simulink model "ddc_bpm_476_066"  (Simulink 7.8)
settings: Solver=ode45  StartTime=0.0  StopTime=4e-4  RelTol=1e-3
undefined symbols (not defined in the file): dt_sim, frev_476, Fs_adc, xlipgetpartsetting
libraries: xbsIndex_r4 x515, simulink x3
(part 4 of 6)

== system ddc_bpm_476_066/Channel0_fofb/Analysis ==
  CIC_FOFB : Scope  NumInputPorts=2
      settings: TimeRange=0.00011214  YMin=-0.232331~-0.265937  YMax=-0.232331~-0.265937  SaveName=ScopeData4  MaxDataPoints=1000000  SampleInput=on
  CORDIC_FOFB : Scope  NumInputPorts=2
      settings: TimeRange=0.00011214  YMin=0.475054~-10  YMax=0.52506~45  SaveName=ScopeData5  MaxDataPoints=1000000  SampleInput=on
  bpf_ch0_o{5..8} (4 alike) : xbsIndex_r4/Gateway Out  inherit_from_input=on  hdl_port=off  timing_constraint=Data Rate  locs_specified=off  LOCs={}  UseAsDAC=off  DACChannel='1'  block_type=gatewayout
      settings: infoedit="Gateway out block.  Converts Xilinx fixed-point or floating-point type inputs into ouputs of type Simulink integer, single, double, or fixed point.<br><br>Hardware notes:  In hardware these blocks become top level output ports or are discarded, depending on how they are configured."
  wires:
  bpf_ch0_o5/1 -> CIC_FOFB/1
  [CIC_FOFB_I_FPGA_OUT] -> bpf_ch0_o5/1
  bpf_ch0_o6/1 -> CIC_FOFB/2
  [CIC_FOFB_Q_FPGA_OUT] -> bpf_ch0_o6/1
  bpf_ch0_o7/1 -> CORDIC_FOFB/1
  [CORDIC_FOFB_R_FPGA_OUT] -> bpf_ch0_o7/1
  bpf_ch0_o8/1 -> CORDIC_FOFB/2
  [CORDIC_FOFB_T_FPGA_OUT] -> bpf_ch0_o8/1

== system ddc_bpm_476_066/Channel0_fofb/cic_fofb ==
  Q_in : Inport
  I_in : Inport  Port=2
  Reinterpret : xbsIndex_r4/Reinterpret  force_arith_type=on  arith_type="Signed  (2's comp)"  force_bin_pt=on  bin_pt=23  block_type=reinterpret
  Reinterpret1 : xbsIndex_r4/Reinterpret  force_arith_type=on  arith_type="Signed  (2's comp)"  force_bin_pt=on  bin_pt=23  block_type=reinterpret
  Terminator : Terminator
  Terminator1 : Terminator
  cic_fofb_i : xbsIndex_r4/CIC Compiler 3.0   filter_type=Decimation  number_of_stages=5  differential_delay=2  number_of_channels=1  sample_rate_changes=Fixed  fixed_or_initial_rate=R_fofb  minimum_rate=1113  maximum_rate=1113  ratespecification=Maximum_Possible  sampleperiod=1  hardwareoversamplingrate=1  quantization=Truncation  output_data_width=25  use_xtreme_dsp_slice=on  use_streaming_interface=on  has_aclken=off  has_aresetn=off  has_dout_tready=off  trim_axipin_name=on  gui_behaviour=Sysgen_GUI  input_data_width=18  ip_name=CIC Compiler  ip_version=3.0  dsptool_ready=true  wrapper_available=true  port_translation_map={ 'aclken' => 'en', 'aresetn' => 'rst' }  ipcore_xco_need_fpga_part=true  ipcore_fpga_part=xlipgetpartsetting(gcb, {'virtex7', 'xc7v1500t', '-2', 'fhg1157'})  ipcore_verbose=false  block_type=cic_compiler_v3_0
  cic_fofb_q : xbsIndex_r4/CIC Compiler 3.0   filter_type=Decimation  number_of_stages=5  differential_delay=2  number_of_channels=1  sample_rate_changes=Fixed  fixed_or_initial_rate=R_fofb  minimum_rate=1113  maximum_rate=1113  ratespecification=Maximum_Possible  sampleperiod=1  hardwareoversamplingrate=1  quantization=Truncation  output_data_width=25  use_xtreme_dsp_slice=on  use_streaming_interface=on  has_aclken=off  has_aresetn=off  has_dout_tready=off  trim_axipin_name=on  gui_behaviour=Sysgen_GUI  input_data_width=18  ip_name=CIC Compiler  ip_version=3.0  dsptool_ready=true  wrapper_available=true  port_translation_map={ 'aclken' => 'en', 'aresetn' => 'rst' }  ipcore_xco_need_fpga_part=true  ipcore_fpga_part=xlipgetpartsetting(gcb, {'virtex7', 'xc7v1500t', '-2', 'fhg1157'})  ipcore_verbose=false  block_type=cic_compiler_v3_0
  Q_out : Outport
  Q_valid : Outport  Port=2
  I_out : Outport  Port=3
  I_valid : Outport  Port=4
  wires:
  I_in/1 -> cic_fofb_i/1
  cic_fofb_i/2 -> I_valid/1
  Q_in/1 -> cic_fofb_q/1
  cic_fofb_q/2 -> Q_valid/1
  cic_fofb_i/1 -> Terminator/1
  cic_fofb_q/1 -> Terminator1/1
  Reinterpret/1 -> Q_out/1
  cic_fofb_q/3 -> Reinterpret/1
  Reinterpret1/1 -> I_out/1
  cic_fofb_i/3 -> Reinterpret1/1

== system ddc_bpm_476_066/Channel0_tbt/Analysis ==
  ADC_in1 : Scope
      settings: TimeRange=0.00011214  YMin=-0.1  YMax=0.1  MaxDataPoints=1000000  SampleInput=on
  ADC_in_FPGA : Scope
      settings: TimeRange=0.00011214  YMin=-0.25  YMax=0.25  SaveName=ScopeData3  MaxDataPoints=1000000  SampleInput=on
  BPF_ADC : Scope
      settings: TimeRange=0.00011214  YMin=-0.25  YMax=0.25  MaxDataPoints=1000000  SampleInput=on
  CORDIC : Scope  NumInputPorts=2
      settings: TimeRange=0.00011214  YMin=0.475054~-10  YMax=0.52506~45  SaveName=ScopeData5  MaxDataPoints=1000000  SampleInput=on
  DECIM_35 : Scope  NumInputPorts=2
      settings: TimeRange=0.00011214  YMin=0.440352~-0.0607492  YMax=0.440353~-0.060745  SaveName=ScopeData4  MaxDataPoints=1000000  SampleInput=on
  Gateway Out : xbsIndex_r4/Gateway Out  inherit_from_input=on  hdl_port=off  timing_constraint=None  locs_specified=off  LOCs={}  UseAsDAC=off  DACChannel='1'  block_type=gatewayout
      settings: infoedit="Gateway out block.  Converts Xilinx fixed-point or floating-point type inputs into ouputs of type Simulink integer, single, double, or fixed point.<br><br>Hardware notes:  In hardware these blocks become top level output ports or are discarded, depending on how they are configured."
  Gateway Out1 : xbsIndex_r4/Gateway Out  inherit_from_input=on  hdl_port=off  timing_constraint=None  locs_specified=off  LOCs={}  UseAsDAC=off  DACChannel='1'  block_type=gatewayout
      settings: infoedit="Gateway out block.  Converts Xilinx fixed-point or floating-point type inputs into ouputs of type Simulink integer, single, double, or fixed point.<br><br>Hardware notes:  In hardware these blocks become top level output ports or are discarded, depending on how they are configured."
  MIX : Scope  NumInputPorts=4
      settings: TimeRange=0.00011214  YMin=-0.1~-1.5~-0.002~-1.5  YMax=1~1.5~0.00075~1.5  SaveName=ScopeData2  MaxDataPoints=1000000  SampleInput=on
  bpf_ch0_o{3..10} (8 alike) : xbsIndex_r4/Gateway Out  inherit_from_input=on  hdl_port=off  timing_constraint=Data Rate  locs_specified=off  LOCs={}  UseAsDAC=off  DACChannel='1'  block_type=gatewayout
      settings: infoedit="Gateway out block.  Converts Xilinx fixed-point or floating-point type inputs into ouputs of type Simulink integer, single, double, or fixed point.<br><br>Hardware notes:  In hardware these blocks become top level output ports or are discarded, depending on how they are configured."
  wires:
  [BPF_ADC_FPGA_OUT] -> Gateway Out1/1
  [ADC_IN] -> ADC_in1/1
  [ADC_IN_FPGA] -> Gateway Out/1
  Gateway Out1/1 -> BPF_ADC/1
  Gateway Out/1 -> ADC_in_FPGA/1
  bpf_ch0_o3/1 -> MIX/1
  [MIX_I_FPGA_OUT] -> bpf_ch0_o3/1
  [MIX_Q_FPGA_OUT] -> bpf_ch0_o4/1
  bpf_ch0_o4/1 -> MIX/3
  [DDS_MSIN_FPGA_OUT] -> bpf_ch0_o9/1
  bpf_ch0_o9/1 -> MIX/2
  [DDS_COS_FPGA_OUT] -> bpf_ch0_o10/1
  bpf_ch0_o10/1 -> MIX/4
  bpf_ch0_o5/1 -> DECIM_35/1
  [DECIM_35_I_FPGA_OUT] -> bpf_ch0_o5/1
  bpf_ch0_o6/1 -> DECIM_35/2
  [DECIM_35_Q_FPGA_OUT] -> bpf_ch0_o6/1
  bpf_ch0_o7/1 -> CORDIC/1
  [CORDIC_R_FPGA_OUT] -> bpf_ch0_o7/1
  bpf_ch0_o8/1 -> CORDIC/2
  [CORDIC_T_FPGA_OUT] -> bpf_ch0_o8/1

== system ddc_bpm_476_066/Channel0_tbt/DDC ==
  adc_in : Inport
  DDS_valid_in : Inport  Port=2
  DDS_msine_in : Inport  Port=3
  DDS_cosine_in : Inport  Port=4
  BPF_FPGA : xbsIndex_r4/FIR Compiler 6.3   coefficientvector=Hbpf_adc.Numerator  coefficient_sets=1  coefficient_reload=off  filter_type=Single_Rate  rate_change_type=Integer  interpolation_rate=1  decimation_rate=1  zero_pack_factor=1  channel_sequence=Basic  number_channels=1  pattern_list='P4-0,P4-1,P4-2,P4-3,P4-4'  number_paths=1  ratespecification=Hardware_Oversampling_Rate  sampleperiod=94  hardwareoversamplingrate=1  coefficient_sign=Signed  quantization=Quantize_Only  coefficient_width=16  bestprecision=off  coefficient_fractional_bits=17  coefficient_structure=Inferred  output_rounding_mode=Full_Precision  output_width=34  filter_architecture=Systolic_Multiply_Accumulate  optimization_goal=Area  data_buffer_type=Automatic  coefficient_buffer_type=Automatic  input_buffer_type=Automatic  output_buffer_type=Automatic  preference_for_other_storage=Automatic  multi_column_support=Automatic  columnconfig='41'  inter_column_pipe_length=4  data_has_tlast=Not_Required  m_data_has_tready=off  s_data_has_fifo=off  s_data_has_tuser=Not_Required  m_data_has_tuser=Not_Required  s_config_sync_mode=On_Vector  s_config_method=Single  num_reload_slots=1  has_aclken=off  has_aresetn=off  infoeditControl=ARESETn must be asserted for a minmum of 2 cycles  trim_axipin_name=on  passband_min=0.0  passband_max=0.5  stopband_min=0.5  stopband_max=1.0  filter_selection=1  gui_behaviour=Sysgen_GUI  data_sign=Signed  data_width=16  data_fractional_bits=0  data_tuser_width=1  wrapper_available=true  ip_wrap_arbitrary_binary_point=true  simulation_type=external_xfix  simulation_model=firv6_3_CModel:firv6_3_cmodel  ip_name=FIR Compiler  ip_version=6.3  dsptool_ready=true  ipcore_usecache=true  ipcore_useipmodelcache=true  ipcore_xco_need_fpga_part=true  port_translation_map={ 'aclken' => 'en', 'aresetn' => 'rst' }  run_core_at_system_period=true  ipcore_fpga_part=xlipgetpartsetting(gcb, {'virtex6', 'xc6vlx75t', '-3', 'ff784'})  block_type=fir_compiler_v6_3
      settings: infoedit=Maximum Possible : Maximizes oversampling rate. Abstracted input handshake (no s_data_tvalid) and automatic rate propagation.<br>Hardware Oversampling Rate : Specifies oversampling rate relative to the input sample period. Abstracted input handshake (no s_data_tvalid) and automatic rate propagation.<br>Sample Period : Specifies absolute oversampling rate. No input handshake abstraction (exposes s_data_tvalid) and no rate propagation.
  Constant1 : xbsIndex_r4/Constant  const=1  gui_display_data_type=Boolean  arith_type=Boolean  n_bits=24  bin_pt=22  preci_type=Single  exp_width=8  frac_width=24  explicit_period=on  period=dt_sim  equ=P=C  opselect=C  inp2=PCIN>>17  opr=+  inp1=P  carry=CIN  dbl_ovrd=off  block_type=constant
  Constant2 : xbsIndex_r4/Constant  const=0  gui_display_data_type=Fixed-point  arith_type=Signed (2's comp)  n_bits=24  bin_pt=22  preci_type=Single  exp_width=8  frac_width=24  explicit_period=on  period=dt_sim  equ=P=C  opselect=C  inp2=PCIN>>17  opr=+  inp1=P  carry=CIN  dbl_ovrd=off  block_type=constant
  Convert : xbsIndex_r4/Convert  gui_display_data_type=Fixed-point  arith_type="Signed  (2's comp)"  n_bits=24  bin_pt=22  float_type=Single  exp_bits=8  fraction_bits=24  quantization=Truncate  overflow=Flag as error  en=off  latency=0  dbl_ovrd=off  pipeline=off  block_type=convert
  DataReg_En : Subsystem
  Mixer : Subsystem
  Register : xbsIndex_r4/Register  init=0  rst=off  en=off  dbl_ovrd=off  block_type=register
  Terminator : Terminator
  Terminator2 : Terminator
  bpf_out : Outport
  mix_q_out : Outport  Port=2
  mix_i_out : Outport  Port=3
  valid_out : Outport  Port=4
  wires:
  Register/1 -> BPF_FPGA/1
  Constant1/1 -> Mixer/3(en)
  Constant2/1 -> Mixer/1(din_q)
  DDS_valid_in/1 -> Mixer/4(dds_valid)
  DDS_cosine_in/1 -> Mixer/5(dds_cosine)
  DDS_msine_in/1 -> Mixer/6(dds_msine)
  BPF_FPGA/3 -> Convert/1
  Convert/1 -> DataReg_En/1(Din)
  DataReg_En/1(Dout) -> Mixer/2(din_i), bpf_out/1
  BPF_FPGA/2 -> DataReg_En/2(en)
  DataReg_En/2(Valid) -> Terminator2/1
  BPF_FPGA/1 -> Terminator/1
  adc_in/1 -> Register/1
  Mixer/1(Q) -> mix_q_out/1
  Mixer/2(I) -> mix_i_out/1
  Mixer/3(valid_out) -> valid_out/1

== system ddc_bpm_476_066/Channel0_tbt/decim35 ==
  Q_in : Inport
  I_in : Inport  Port=2
  Convert1 : xbsIndex_r4/Convert  gui_display_data_type=Fixed-point  arith_type="Signed  (2's comp)"  n_bits=25  bin_pt=23  float_type=Single  exp_bits=8  fraction_bits=24  quantization="Round  (unbiased: +/- Inf)"  overflow=Flag as error  en=off  latency=0  dbl_ovrd=off  pipeline=off  block_type=convert
  Convert2 : xbsIndex_r4/Convert  gui_display_data_type=Fixed-point  arith_type="Signed  (2's comp)"  n_bits=25  bin_pt=23  float_type=Single  exp_bits=8  fraction_bits=24  quantization="Round  (unbiased: +/- Inf)"  overflow=Flag as error  en=off  latency=0  dbl_ovrd=off  pipeline=off  block_type=convert
  "FIR Compiler 6.2 " : xbsIndex_r4/FIR Compiler 6.2   coefficientvector=Hpoly_35.Numerator  coefficient_sets=1  filter_type=Decimation  rate_change_type=Integer  interpolation_rate=1  decimation_rate=decim_factor_poly_35  number_channels=1  ratespecification=Maximum_Possible  sampleperiod=1  hardwareoversamplingrate=1  filter_architecture=Systolic_Multiply_Accumulate  coefficient_reload=off  coefficient_sign=Signed  quantization=Quantize_Only  coefficient_width=16  bestprecision=on  coefficient_fractional_bits=20  coefficient_structure=Inferred  number_paths=2  output_rounding_mode=Full_Precision  output_width=37  optimization_goal=Area  data_has_tlast=Not_Required  m_data_has_tready=off  s_data_has_fifo=off  s_data_has_tuser=Not_Required  m_data_has_tuser=Not_Required  s_config_sync_mode=On_Vector  s_config_method=Single  num_reload_slots=1  has_aclken=off  has_aresetn=off  multi_column_support=Disabled  columnconfig='14'  inter_column_pipe_length=4  data_buffer_type=Automatic  coefficient_buffer_type=Automatic  input_buffer_type=Automatic  output_buffer_type=Automatic  preference_for_other_storage=Automatic  trim_axipin_name=on  passband_min=0.0  passband_max=0.5  stopband_min=0.5  stopband_max=1.0  filter_selection=1  gui_behaviour=Sysgen_GUI  data_sign=Signed  data_width=16  data_fractional_bits=0  wrapper_available=true  ip_wrap_arbitrary_binary_point=true  ip_name=FIR Compiler  ip_version=6.2  dsptool_ready=true  ipcore_usecache=true  ipcore_useipmodelcache=true  ipcore_xco_need_fpga_part=true  port_translation_map={ 'aclken' => 'en', 'aresetn' => 'rst' }  run_core_at_system_period=true  ipcore_fpga_part=xlipgetpartsetting(gcb, {'virtex6', 'xc6vlx75t', '-3', 'ff784'})  structural_sim=false  block_type=fir_compiler_v6_2
      settings: infoedit=Maximum Possible : Maximizes oversampling rate. Abstracted input handshake (no s_data_tvalid) and automatic rate propagation.<br>Hardware Oversampling Rate : Specifies oversampling rate relative to the input sample period. Abstracted input handshake (no s_data_tvalid) and automatic rate propagation.<br>Sample Period : Specifies absolute oversampling rate. No input handshake abstraction (exposes s_data_tvalid) and no rate propagation.
  Reinterpret : xbsIndex_r4/Reinterpret  force_arith_type=off  arith_type=Unsigned  force_bin_pt=off  bin_pt=43  block_type=reinterpret
  Reinterpret1 : xbsIndex_r4/Reinterpret  force_arith_type=off  arith_type=Unsigned  force_bin_pt=off  bin_pt=43  block_type=reinterpret
  Terminator : Terminator
  Q_out : Outport
  I_out : Outport  Port=2
  valid_out : Outport  Port=3
  wires:
  Q_in/1 -> "FIR Compiler 6.2 "/1
  "FIR Compiler 6.2 "/2 -> valid_out/1
  Reinterpret/1 -> Convert1/1
  "FIR Compiler 6.2 "/3 -> Reinterpret/1
  Convert1/1 -> Q_out/1
  Reinterpret1/1 -> Convert2/1
  "FIR Compiler 6.2 "/4 -> Reinterpret1/1
  Convert2/1 -> I_out/1
  I_in/1 -> "FIR Compiler 6.2 "/2
  "FIR Compiler 6.2 "/1 -> Terminator/1

== system ddc_bpm_476_066/Channel1_fofb/Analysis ==
  CIC_FOFB : Scope  NumInputPorts=2
      settings: TimeRange=0.00011214  YMin=0.440352~-0.0607492  YMax=0.440353~-0.060745  SaveName=ScopeData4  MaxDataPoints=1000000  SampleInput=on
  CORDIC_FOFB : Scope  NumInputPorts=2
      settings: TimeRange=0.00011214  YMin=0.475054~-10  YMax=0.52506~45  SaveName=ScopeData5  MaxDataPoints=1000000  SampleInput=on
  bpf_ch0_o{5..8} (4 alike) : xbsIndex_r4/Gateway Out  inherit_from_input=on  hdl_port=off  timing_constraint=Data Rate  locs_specified=off  LOCs={}  UseAsDAC=off  DACChannel='1'  block_type=gatewayout
      settings: infoedit="Gateway out block.  Converts Xilinx fixed-point or floating-point type inputs into ouputs of type Simulink integer, single, double, or fixed point.<br><br>Hardware notes:  In hardware these blocks become top level output ports or are discarded, depending on how they are configured."
  wires:
  bpf_ch0_o5/1 -> CIC_FOFB/1
  [CIC_FOFB_I_FPGA_OUT] -> bpf_ch0_o5/1
  bpf_ch0_o6/1 -> CIC_FOFB/2
  [CIC_FOFB_Q_FPGA_OUT] -> bpf_ch0_o6/1
  bpf_ch0_o7/1 -> CORDIC_FOFB/1
  [CORDIC_FOFB_R_FPGA_OUT] -> bpf_ch0_o7/1
  bpf_ch0_o8/1 -> CORDIC_FOFB/2
  [CORDIC_FOFB_T_FPGA_OUT] -> bpf_ch0_o8/1

== system ddc_bpm_476_066/Channel1_fofb/cic_fofb ==
  Q_in : Inport
  I_in : Inport  Port=2
  Reinterpret : xbsIndex_r4/Reinterpret  force_arith_type=on  arith_type="Signed  (2's comp)"  force_bin_pt=on  bin_pt=23  block_type=reinterpret
  Reinterpret1 : xbsIndex_r4/Reinterpret  force_arith_type=on  arith_type="Signed  (2's comp)"  force_bin_pt=on  bin_pt=23  block_type=reinterpret
  Terminator : Terminator
  Terminator1 : Terminator
  cic_fofb_i : xbsIndex_r4/CIC Compiler 3.0   filter_type=Decimation  number_of_stages=5  differential_delay=2  number_of_channels=1  sample_rate_changes=Fixed  fixed_or_initial_rate=R_fofb  minimum_rate=1113  maximum_rate=1113  ratespecification=Maximum_Possible  sampleperiod=1  hardwareoversamplingrate=1  quantization=Truncation  output_data_width=25  use_xtreme_dsp_slice=on  use_streaming_interface=on  has_aclken=off  has_aresetn=off  has_dout_tready=off  trim_axipin_name=on  gui_behaviour=Sysgen_GUI  input_data_width=18  ip_name=CIC Compiler  ip_version=3.0  dsptool_ready=true  wrapper_available=true  port_translation_map={ 'aclken' => 'en', 'aresetn' => 'rst' }  ipcore_xco_need_fpga_part=true  ipcore_fpga_part=xlipgetpartsetting(gcb, {'virtex7', 'xc7v1500t', '-2', 'fhg1157'})  ipcore_verbose=false  block_type=cic_compiler_v3_0
  cic_fofb_q : xbsIndex_r4/CIC Compiler 3.0   filter_type=Decimation  number_of_stages=5  differential_delay=2  number_of_channels=1  sample_rate_changes=Fixed  fixed_or_initial_rate=R_fofb  minimum_rate=1113  maximum_rate=1113  ratespecification=Maximum_Possible  sampleperiod=1  hardwareoversamplingrate=1  quantization=Truncation  output_data_width=25  use_xtreme_dsp_slice=on  use_streaming_interface=on  has_aclken=off  has_aresetn=off  has_dout_tready=off  trim_axipin_name=on  gui_behaviour=Sysgen_GUI  input_data_width=18  ip_name=CIC Compiler  ip_version=3.0  dsptool_ready=true  wrapper_available=true  port_translation_map={ 'aclken' => 'en', 'aresetn' => 'rst' }  ipcore_xco_need_fpga_part=true  ipcore_fpga_part=xlipgetpartsetting(gcb, {'virtex7', 'xc7v1500t', '-2', 'fhg1157'})  ipcore_verbose=false  block_type=cic_compiler_v3_0
  Q_out : Outport
  Q_valid : Outport  Port=2
  I_out : Outport  Port=3
  I_valid : Outport  Port=4
  wires:
  I_in/1 -> cic_fofb_i/1
  cic_fofb_i/2 -> I_valid/1
  Q_in/1 -> cic_fofb_q/1
  cic_fofb_q/2 -> Q_valid/1
  cic_fofb_i/1 -> Terminator/1
  cic_fofb_q/1 -> Terminator1/1
  Reinterpret/1 -> Q_out/1
  cic_fofb_q/3 -> Reinterpret/1
  Reinterpret1/1 -> I_out/1
  cic_fofb_i/3 -> Reinterpret1/1

== system ddc_bpm_476_066/Channel1_tbt/Analysis ==
  ADC_in1 : Scope
      settings: TimeRange=0.00011214  YMin=-0.1  YMax=0.1  MaxDataPoints=1000000  SampleInput=on
  ADC_in_FPGA : Scope
      settings: TimeRange=0.00011214  YMin=-0.25  YMax=0.25  SaveName=ScopeData3  MaxDataPoints=1000000  SampleInput=on
  BPF_ADC : Scope
      settings: TimeRange=0.00011214  YMin=-0.25  YMax=0.25  MaxDataPoints=1000000  SampleInput=on
  CORDIC : Scope  NumInputPorts=2
      settings: TimeRange=0.00011214  YMin=0.475054~-10  YMax=0.52506~45  SaveName=ScopeData5  MaxDataPoints=1000000  SampleInput=on
  DECIM_35 : Scope  NumInputPorts=2
      settings: TimeRange=0.00011214  YMin=0.440352~-0.0607492  YMax=0.440353~-0.060745  SaveName=ScopeData4  MaxDataPoints=1000000  SampleInput=on
  Gateway Out : xbsIndex_r4/Gateway Out  inherit_from_input=on  hdl_port=off  timing_constraint=None  locs_specified=off  LOCs={}  UseAsDAC=off  DACChannel='1'  block_type=gatewayout
      settings: infoedit="Gateway out block.  Converts Xilinx fixed-point or floating-point type inputs into ouputs of type Simulink integer, single, double, or fixed point.<br><br>Hardware notes:  In hardware these blocks become top level output ports or are discarded, depending on how they are configured."
  Gateway Out1 : xbsIndex_r4/Gateway Out  inherit_from_input=on  hdl_port=off  timing_constraint=None  locs_specified=off  LOCs={}  UseAsDAC=off  DACChannel='1'  block_type=gatewayout
      settings: infoedit="Gateway out block.  Converts Xilinx fixed-point or floating-point type inputs into ouputs of type Simulink integer, single, double, or fixed point.<br><br>Hardware notes:  In hardware these blocks become top level output ports or are discarded, depending on how they are configured."
  MIX : Scope  NumInputPorts=4
      settings: TimeRange=0.00011214  YMin=-0.1~-1.5~-0.002~-1.5  YMax=1~1.5~0.00075~1.5  SaveName=ScopeData2  MaxDataPoints=1000000  SampleInput=on
  bpf_ch0_o{3..10} (8 alike) : xbsIndex_r4/Gateway Out  inherit_from_input=on  hdl_port=off  timing_constraint=Data Rate  locs_specified=off  LOCs={}  UseAsDAC=off  DACChannel='1'  block_type=gatewayout
      settings: infoedit="Gateway out block.  Converts Xilinx fixed-point or floating-point type inputs into ouputs of type Simulink integer, single, double, or fixed point.<br><br>Hardware notes:  In hardware these blocks become top level output ports or are discarded, depending on how they are configured."
  wires:
  [BPF_ADC_FPGA_OUT] -> Gateway Out1/1
  [ADC_IN] -> ADC_in1/1
  [ADC_IN_FPGA] -> Gateway Out/1
  Gateway Out1/1 -> BPF_ADC/1
  Gateway Out/1 -> ADC_in_FPGA/1
  bpf_ch0_o3/1 -> MIX/1
  [MIX_I_FPGA_OUT] -> bpf_ch0_o3/1
  [MIX_Q_FPGA_OUT] -> bpf_ch0_o4/1
  bpf_ch0_o4/1 -> MIX/3
  [DDS_MSIN_FPGA_OUT] -> bpf_ch0_o9/1
  bpf_ch0_o9/1 -> MIX/2
  [DDS_COS_FPGA_OUT] -> bpf_ch0_o10/1
  bpf_ch0_o10/1 -> MIX/4
  bpf_ch0_o5/1 -> DECIM_35/1
  [DECIM_35_I_FPGA_OUT] -> bpf_ch0_o5/1
  bpf_ch0_o6/1 -> DECIM_35/2
  [DECIM_35_Q_FPGA_OUT] -> bpf_ch0_o6/1
  bpf_ch0_o7/1 -> CORDIC/1
  [CORDIC_R_FPGA_OUT] -> bpf_ch0_o7/1
  bpf_ch0_o8/1 -> CORDIC/2
  [CORDIC_T_FPGA_OUT] -> bpf_ch0_o8/1

== system ddc_bpm_476_066/Channel1_tbt/DDC ==
  adc_in : Inport
  DDS_valid_in : Inport  Port=2
  DDS_msine_in : Inport  Port=3
  DDS_cosine_in : Inport  Port=4
  BPF_FPGA : xbsIndex_r4/FIR Compiler 6.3   coefficientvector=Hbpf_adc.Numerator  coefficient_sets=1  coefficient_reload=off  filter_type=Single_Rate  rate_change_type=Integer  interpolation_rate=1  decimation_rate=1  zero_pack_factor=1  channel_sequence=Basic  number_channels=1  pattern_list='P4-0,P4-1,P4-2,P4-3,P4-4'  number_paths=1  ratespecification=Hardware_Oversampling_Rate  sampleperiod=94  hardwareoversamplingrate=1  coefficient_sign=Signed  quantization=Quantize_Only  coefficient_width=16  bestprecision=off  coefficient_fractional_bits=17  coefficient_structure=Inferred  output_rounding_mode=Full_Precision  output_width=34  filter_architecture=Systolic_Multiply_Accumulate  optimization_goal=Area  data_buffer_type=Automatic  coefficient_buffer_type=Automatic  input_buffer_type=Automatic  output_buffer_type=Automatic  preference_for_other_storage=Automatic  multi_column_support=Automatic  columnconfig='41'  inter_column_pipe_length=4  data_has_tlast=Not_Required  m_data_has_tready=off  s_data_has_fifo=off  s_data_has_tuser=Not_Required  m_data_has_tuser=Not_Required  s_config_sync_mode=On_Vector  s_config_method=Single  num_reload_slots=1  has_aclken=off  has_aresetn=off  infoeditControl=ARESETn must be asserted for a minmum of 2 cycles  trim_axipin_name=on  passband_min=0.0  passband_max=0.5  stopband_min=0.5  stopband_max=1.0  filter_selection=1  gui_behaviour=Sysgen_GUI  data_sign=Signed  data_width=16  data_fractional_bits=0  data_tuser_width=1  wrapper_available=true  ip_wrap_arbitrary_binary_point=true  simulation_type=external_xfix  simulation_model=firv6_3_CModel:firv6_3_cmodel  ip_name=FIR Compiler  ip_version=6.3  dsptool_ready=true  ipcore_usecache=true  ipcore_useipmodelcache=true  ipcore_xco_need_fpga_part=true  port_translation_map={ 'aclken' => 'en', 'aresetn' => 'rst' }  run_core_at_system_period=true  ipcore_fpga_part=xlipgetpartsetting(gcb, {'virtex6', 'xc6vlx75t', '-3', 'ff784'})  block_type=fir_compiler_v6_3
      settings: infoedit=Maximum Possible : Maximizes oversampling rate. Abstracted input handshake (no s_data_tvalid) and automatic rate propagation.<br>Hardware Oversampling Rate : Specifies oversampling rate relative to the input sample period. Abstracted input handshake (no s_data_tvalid) and automatic rate propagation.<br>Sample Period : Specifies absolute oversampling rate. No input handshake abstraction (exposes s_data_tvalid) and no rate propagation.
  Constant1 : xbsIndex_r4/Constant  const=1  gui_display_data_type=Boolean  arith_type=Boolean  n_bits=24  bin_pt=22  preci_type=Single  exp_width=8  frac_width=24  explicit_period=on  period=dt_sim  equ=P=C  opselect=C  inp2=PCIN>>17  opr=+  inp1=P  carry=CIN  dbl_ovrd=off  block_type=constant
  Constant2 : xbsIndex_r4/Constant  const=0  gui_display_data_type=Fixed-point  arith_type=Signed (2's comp)  n_bits=24  bin_pt=22  preci_type=Single  exp_width=8  frac_width=24  explicit_period=on  period=dt_sim  equ=P=C  opselect=C  inp2=PCIN>>17  opr=+  inp1=P  carry=CIN  dbl_ovrd=off  block_type=constant
  Convert : xbsIndex_r4/Convert  gui_display_data_type=Fixed-point  arith_type="Signed  (2's comp)"  n_bits=24  bin_pt=22  float_type=Single  exp_bits=8  fraction_bits=24  quantization=Truncate  overflow=Flag as error  en=off  latency=0  dbl_ovrd=off  pipeline=off  block_type=convert
  DataReg_En : Subsystem
  Mixer : Subsystem
  Register : xbsIndex_r4/Register  init=0  rst=off  en=off  dbl_ovrd=off  block_type=register
  Terminator : Terminator
  Terminator2 : Terminator
  bpf_out : Outport
  mix_q_out : Outport  Port=2
  mix_i_out : Outport  Port=3
  valid_out : Outport  Port=4
  wires:
  Register/1 -> BPF_FPGA/1
  Constant1/1 -> Mixer/3(en)
  Constant2/1 -> Mixer/1(din_q)
  DDS_valid_in/1 -> Mixer/4(dds_valid)
  DDS_cosine_in/1 -> Mixer/5(dds_cosine)
  DDS_msine_in/1 -> Mixer/6(dds_msine)
  BPF_FPGA/3 -> Convert/1
  Convert/1 -> DataReg_En/1(Din)
  DataReg_En/1(Dout) -> Mixer/2(din_i), bpf_out/1
  BPF_FPGA/2 -> DataReg_En/2(en)
  DataReg_En/2(Valid) -> Terminator2/1
  BPF_FPGA/1 -> Terminator/1
  adc_in/1 -> Register/1
  Mixer/1(Q) -> mix_q_out/1
  Mixer/2(I) -> mix_i_out/1
  Mixer/3(valid_out) -> valid_out/1

== system ddc_bpm_476_066/Channel1_tbt/decim35 ==
  Q_in : Inport
  I_in : Inport  Port=2
  Convert1 : xbsIndex_r4/Convert  gui_display_data_type=Fixed-point  arith_type="Signed  (2's comp)"  n_bits=25  bin_pt=23  float_type=Single  exp_bits=8  fraction_bits=24  quantization="Round  (unbiased: +/- Inf)"  overflow=Flag as error  en=off  latency=0  dbl_ovrd=off  pipeline=off  block_type=convert
  Convert2 : xbsIndex_r4/Convert  gui_display_data_type=Fixed-point  arith_type="Signed  (2's comp)"  n_bits=25  bin_pt=23  float_type=Single  exp_bits=8  fraction_bits=24  quantization="Round  (unbiased: +/- Inf)"  overflow=Flag as error  en=off  latency=0  dbl_ovrd=off  pipeline=off  block_type=convert
  "FIR Compiler 6.2 " : xbsIndex_r4/FIR Compiler 6.2   coefficientvector=Hpoly_35.Numerator  coefficient_sets=1  filter_type=Decimation  rate_change_type=Integer  interpolation_rate=1  decimation_rate=decim_factor_poly_35  number_channels=1  ratespecification=Maximum_Possible  sampleperiod=1  hardwareoversamplingrate=1  filter_architecture=Systolic_Multiply_Accumulate  coefficient_reload=off  coefficient_sign=Signed  quantization=Quantize_Only  coefficient_width=16  bestprecision=on  coefficient_fractional_bits=20  coefficient_structure=Inferred  number_paths=2  output_rounding_mode=Full_Precision  output_width=37  optimization_goal=Area  data_has_tlast=Not_Required  m_data_has_tready=off  s_data_has_fifo=off  s_data_has_tuser=Not_Required  m_data_has_tuser=Not_Required  s_config_sync_mode=On_Vector  s_config_method=Single  num_reload_slots=1  has_aclken=off  has_aresetn=off  multi_column_support=Disabled  columnconfig='14'  inter_column_pipe_length=4  data_buffer_type=Automatic  coefficient_buffer_type=Automatic  input_buffer_type=Automatic  output_buffer_type=Automatic  preference_for_other_storage=Automatic  trim_axipin_name=on  passband_min=0.0  passband_max=0.5  stopband_min=0.5  stopband_max=1.0  filter_selection=1  gui_behaviour=Sysgen_GUI  data_sign=Signed  data_width=16  data_fractional_bits=0  wrapper_available=true  ip_wrap_arbitrary_binary_point=true  ip_name=FIR Compiler  ip_version=6.2  dsptool_ready=true  ipcore_usecache=true  ipcore_useipmodelcache=true  ipcore_xco_need_fpga_part=true  port_translation_map={ 'aclken' => 'en', 'aresetn' => 'rst' }  run_core_at_system_period=true  ipcore_fpga_part=xlipgetpartsetting(gcb, {'virtex6', 'xc6vlx75t', '-3', 'ff784'})  structural_sim=false  block_type=fir_compiler_v6_2
      settings: infoedit=Maximum Possible : Maximizes oversampling rate. Abstracted input handshake (no s_data_tvalid) and automatic rate propagation.<br>Hardware Oversampling Rate : Specifies oversampling rate relative to the input sample period. Abstracted input handshake (no s_data_tvalid) and automatic rate propagation.<br>Sample Period : Specifies absolute oversampling rate. No input handshake abstraction (exposes s_data_tvalid) and no rate propagation.
  Reinterpret : xbsIndex_r4/Reinterpret  force_arith_type=off  arith_type=Unsigned  force_bin_pt=off  bin_pt=43  block_type=reinterpret
  Reinterpret1 : xbsIndex_r4/Reinterpret  force_arith_type=off  arith_type=Unsigned  force_bin_pt=off  bin_pt=43  block_type=reinterpret
  Terminator : Terminator
  Q_out : Outport
  I_out : Outport  Port=2
  valid_out : Outport  Port=3
  wires:
  Q_in/1 -> "FIR Compiler 6.2 "/1
  "FIR Compiler 6.2 "/2 -> valid_out/1
  Reinterpret/1 -> Convert1/1
  "FIR Compiler 6.2 "/3 -> Reinterpret/1
  Convert1/1 -> Q_out/1
  Reinterpret1/1 -> Convert2/1
  "FIR Compiler 6.2 "/4 -> Reinterpret1/1
  Convert2/1 -> I_out/1
  I_in/1 -> "FIR Compiler 6.2 "/2
  "FIR Compiler 6.2 "/1 -> Terminator/1

== system ddc_bpm_476_066/Channel2_fofb/Analysis ==
  CIC_FOFB : Scope  NumInputPorts=2
      settings: TimeRange=0.00011214  YMin=0.440352~-0.0607492  YMax=0.440353~-0.060745  SaveName=ScopeData4  MaxDataPoints=1000000  SampleInput=on
  CORDIC_FOFB : Scope  NumInputPorts=2
      settings: TimeRange=0.00011214  YMin=0.475054~-10  YMax=0.52506~45  SaveName=ScopeData5  MaxDataPoints=1000000  SampleInput=on
  bpf_ch0_o{5..8} (4 alike) : xbsIndex_r4/Gateway Out  inherit_from_input=on  hdl_port=off  timing_constraint=Data Rate  locs_specified=off  LOCs={}  UseAsDAC=off  DACChannel='1'  block_type=gatewayout
      settings: infoedit="Gateway out block.  Converts Xilinx fixed-point or floating-point type inputs into ouputs of type Simulink integer, single, double, or fixed point.<br><br>Hardware notes:  In hardware these blocks become top level output ports or are discarded, depending on how they are configured."
  wires:
  bpf_ch0_o5/1 -> CIC_FOFB/1
  [CIC_FOFB_I_FPGA_OUT] -> bpf_ch0_o5/1
  bpf_ch0_o6/1 -> CIC_FOFB/2
  [CIC_FOFB_Q_FPGA_OUT] -> bpf_ch0_o6/1
  bpf_ch0_o7/1 -> CORDIC_FOFB/1
  [CORDIC_FOFB_R_FPGA_OUT] -> bpf_ch0_o7/1
  bpf_ch0_o8/1 -> CORDIC_FOFB/2
  [CORDIC_FOFB_T_FPGA_OUT] -> bpf_ch0_o8/1

== system ddc_bpm_476_066/Channel2_fofb/cic_fofb ==
  Q_in : Inport
  I_in : Inport  Port=2
  Reinterpret : xbsIndex_r4/Reinterpret  force_arith_type=on  arith_type="Signed  (2's comp)"  force_bin_pt=on  bin_pt=23  block_type=reinterpret
  Reinterpret1 : xbsIndex_r4/Reinterpret  force_arith_type=on  arith_type="Signed  (2's comp)"  force_bin_pt=on  bin_pt=23  block_type=reinterpret
  Terminator : Terminator
  Terminator1 : Terminator
  cic_fofb_i : xbsIndex_r4/CIC Compiler 3.0   filter_type=Decimation  number_of_stages=5  differential_delay=2  number_of_channels=1  sample_rate_changes=Fixed  fixed_or_initial_rate=R_fofb  minimum_rate=1113  maximum_rate=1113  ratespecification=Maximum_Possible  sampleperiod=1  hardwareoversamplingrate=1  quantization=Truncation  output_data_width=25  use_xtreme_dsp_slice=on  use_streaming_interface=on  has_aclken=off  has_aresetn=off  has_dout_tready=off  trim_axipin_name=on  gui_behaviour=Sysgen_GUI  input_data_width=18  ip_name=CIC Compiler  ip_version=3.0  dsptool_ready=true  wrapper_available=true  port_translation_map={ 'aclken' => 'en', 'aresetn' => 'rst' }  ipcore_xco_need_fpga_part=true  ipcore_fpga_part=xlipgetpartsetting(gcb, {'virtex7', 'xc7v1500t', '-2', 'fhg1157'})  ipcore_verbose=false  block_type=cic_compiler_v3_0
  cic_fofb_q : xbsIndex_r4/CIC Compiler 3.0   filter_type=Decimation  number_of_stages=5  differential_delay=2  number_of_channels=1  sample_rate_changes=Fixed  fixed_or_initial_rate=R_fofb  minimum_rate=1113  maximum_rate=1113  ratespecification=Maximum_Possible  sampleperiod=1  hardwareoversamplingrate=1  quantization=Truncation  output_data_width=25  use_xtreme_dsp_slice=on  use_streaming_interface=on  has_aclken=off  has_aresetn=off  has_dout_tready=off  trim_axipin_name=on  gui_behaviour=Sysgen_GUI  input_data_width=18  ip_name=CIC Compiler  ip_version=3.0  dsptool_ready=true  wrapper_available=true  port_translation_map={ 'aclken' => 'en', 'aresetn' => 'rst' }  ipcore_xco_need_fpga_part=true  ipcore_fpga_part=xlipgetpartsetting(gcb, {'virtex7', 'xc7v1500t', '-2', 'fhg1157'})  ipcore_verbose=false  block_type=cic_compiler_v3_0
  Q_out : Outport
  Q_valid : Outport  Port=2
  I_out : Outport  Port=3
  I_valid : Outport  Port=4
  wires:
  I_in/1 -> cic_fofb_i/1
  cic_fofb_i/2 -> I_valid/1
  Q_in/1 -> cic_fofb_q/1
  cic_fofb_q/2 -> Q_valid/1
  cic_fofb_i/1 -> Terminator/1
  cic_fofb_q/1 -> Terminator1/1
  Reinterpret/1 -> Q_out/1
  cic_fofb_q/3 -> Reinterpret/1
  Reinterpret1/1 -> I_out/1
  cic_fofb_i/3 -> Reinterpret1/1

== system ddc_bpm_476_066/Channel2_tbt/Analysis ==
  ADC_in1 : Scope
      settings: TimeRange=0.00011214  YMin=-0.1  YMax=0.1  MaxDataPoints=1000000  SampleInput=on
  ADC_in_FPGA : Scope
      settings: TimeRange=0.00011214  YMin=-0.25  YMax=0.25  SaveName=ScopeData3  MaxDataPoints=1000000  SampleInput=on
  BPF_ADC : Scope
      settings: TimeRange=0.00011214  YMin=-0.25  YMax=0.25  MaxDataPoints=1000000  SampleInput=on
  CORDIC : Scope  NumInputPorts=2
      settings: TimeRange=0.00011214  YMin=0.475054~-10  YMax=0.52506~45  SaveName=ScopeData5  MaxDataPoints=1000000  SampleInput=on
  DECIM_35 : Scope  NumInputPorts=2
      settings: TimeRange=0.00011214  YMin=0.440352~-0.0607492  YMax=0.440353~-0.060745  SaveName=ScopeData4  MaxDataPoints=1000000  SampleInput=on
  Gateway Out : xbsIndex_r4/Gateway Out  inherit_from_input=on  hdl_port=off  timing_constraint=None  locs_specified=off  LOCs={}  UseAsDAC=off  DACChannel='1'  block_type=gatewayout
      settings: infoedit="Gateway out block.  Converts Xilinx fixed-point or floating-point type inputs into ouputs of type Simulink integer, single, double, or fixed point.<br><br>Hardware notes:  In hardware these blocks become top level output ports or are discarded, depending on how they are configured."
  Gateway Out1 : xbsIndex_r4/Gateway Out  inherit_from_input=on  hdl_port=off  timing_constraint=None  locs_specified=off  LOCs={}  UseAsDAC=off  DACChannel='1'  block_type=gatewayout
      settings: infoedit="Gateway out block.  Converts Xilinx fixed-point or floating-point type inputs into ouputs of type Simulink integer, single, double, or fixed point.<br><br>Hardware notes:  In hardware these blocks become top level output ports or are discarded, depending on how they are configured."
  MIX : Scope  NumInputPorts=4
      settings: TimeRange=0.00011214  YMin=-0.1~-1.5~-0.002~-1.5  YMax=1~1.5~0.00075~1.5  SaveName=ScopeData2  MaxDataPoints=1000000  SampleInput=on
  bpf_ch0_o{3..10} (8 alike) : xbsIndex_r4/Gateway Out  inherit_from_input=on  hdl_port=off  timing_constraint=Data Rate  locs_specified=off  LOCs={}  UseAsDAC=off  DACChannel='1'  block_type=gatewayout
      settings: infoedit="Gateway out block.  Converts Xilinx fixed-point or floating-point type inputs into ouputs of type Simulink integer, single, double, or fixed point.<br><br>Hardware notes:  In hardware these blocks become top level output ports or are discarded, depending on how they are configured."
  wires:
  [BPF_ADC_FPGA_OUT] -> Gateway Out1/1
  [ADC_IN] -> ADC_in1/1
  [ADC_IN_FPGA] -> Gateway Out/1
  Gateway Out1/1 -> BPF_ADC/1
  Gateway Out/1 -> ADC_in_FPGA/1
  bpf_ch0_o3/1 -> MIX/1
  [MIX_I_FPGA_OUT] -> bpf_ch0_o3/1
  [MIX_Q_FPGA_OUT] -> bpf_ch0_o4/1
  bpf_ch0_o4/1 -> MIX/3
  [DDS_MSIN_FPGA_OUT] -> bpf_ch0_o9/1
  bpf_ch0_o9/1 -> MIX/2
  [DDS_COS_FPGA_OUT] -> bpf_ch0_o10/1
  bpf_ch0_o10/1 -> MIX/4
  bpf_ch0_o5/1 -> DECIM_35/1
  [DECIM_35_I_FPGA_OUT] -> bpf_ch0_o5/1
  bpf_ch0_o6/1 -> DECIM_35/2
  [DECIM_35_Q_FPGA_OUT] -> bpf_ch0_o6/1
  bpf_ch0_o7/1 -> CORDIC/1
  [CORDIC_R_FPGA_OUT] -> bpf_ch0_o7/1
  bpf_ch0_o8/1 -> CORDIC/2
  [CORDIC_T_FPGA_OUT] -> bpf_ch0_o8/1

== system ddc_bpm_476_066/Channel2_tbt/DDC ==
  adc_in : Inport
  DDS_valid_in : Inport  Port=2
  DDS_msine_in : Inport  Port=3
  DDS_cosine_in : Inport  Port=4
  BPF_FPGA : xbsIndex_r4/FIR Compiler 6.3   coefficientvector=Hbpf_adc.Numerator  coefficient_sets=1  coefficient_reload=off  filter_type=Single_Rate  rate_change_type=Integer  interpolation_rate=1  decimation_rate=1  zero_pack_factor=1  channel_sequence=Basic  number_channels=1  pattern_list='P4-0,P4-1,P4-2,P4-3,P4-4'  number_paths=1  ratespecification=Hardware_Oversampling_Rate  sampleperiod=94  hardwareoversamplingrate=1  coefficient_sign=Signed  quantization=Quantize_Only  coefficient_width=16  bestprecision=off  coefficient_fractional_bits=17  coefficient_structure=Inferred  output_rounding_mode=Full_Precision  output_width=34  filter_architecture=Systolic_Multiply_Accumulate  optimization_goal=Area  data_buffer_type=Automatic  coefficient_buffer_type=Automatic  input_buffer_type=Automatic  output_buffer_type=Automatic  preference_for_other_storage=Automatic  multi_column_support=Automatic  columnconfig='41'  inter_column_pipe_length=4  data_has_tlast=Not_Required  m_data_has_tready=off  s_data_has_fifo=off  s_data_has_tuser=Not_Required  m_data_has_tuser=Not_Required  s_config_sync_mode=On_Vector  s_config_method=Single  num_reload_slots=1  has_aclken=off  has_aresetn=off  infoeditControl=ARESETn must be asserted for a minmum of 2 cycles  trim_axipin_name=on  passband_min=0.0  passband_max=0.5  stopband_min=0.5  stopband_max=1.0  filter_selection=1  gui_behaviour=Sysgen_GUI  data_sign=Signed  data_width=16  data_fractional_bits=0  data_tuser_width=1  wrapper_available=true  ip_wrap_arbitrary_binary_point=true  simulation_type=external_xfix  simulation_model=firv6_3_CModel:firv6_3_cmodel  ip_name=FIR Compiler  ip_version=6.3  dsptool_ready=true  ipcore_usecache=true  ipcore_useipmodelcache=true  ipcore_xco_need_fpga_part=true  port_translation_map={ 'aclken' => 'en', 'aresetn' => 'rst' }  run_core_at_system_period=true  ipcore_fpga_part=xlipgetpartsetting(gcb, {'virtex6', 'xc6vlx75t', '-3', 'ff784'})  block_type=fir_compiler_v6_3
      settings: infoedit=Maximum Possible : Maximizes oversampling rate. Abstracted input handshake (no s_data_tvalid) and automatic rate propagation.<br>Hardware Oversampling Rate : Specifies oversampling rate relative to the input sample period. Abstracted input handshake (no s_data_tvalid) and automatic rate propagation.<br>Sample Period : Specifies absolute oversampling rate. No input handshake abstraction (exposes s_data_tvalid) and no rate propagation.
  Constant1 : xbsIndex_r4/Constant  const=1  gui_display_data_type=Boolean  arith_type=Boolean  n_bits=24  bin_pt=22  preci_type=Single  exp_width=8  frac_width=24  explicit_period=on  period=dt_sim  equ=P=C  opselect=C  inp2=PCIN>>17  opr=+  inp1=P  carry=CIN  dbl_ovrd=off  block_type=constant
  Constant2 : xbsIndex_r4/Constant  const=0  gui_display_data_type=Fixed-point  arith_type=Signed (2's comp)  n_bits=24  bin_pt=22  preci_type=Single  exp_width=8  frac_width=24  explicit_period=on  period=dt_sim  equ=P=C  opselect=C  inp2=PCIN>>17  opr=+  inp1=P  carry=CIN  dbl_ovrd=off  block_type=constant
  Convert : xbsIndex_r4/Convert  gui_display_data_type=Fixed-point  arith_type="Signed  (2's comp)"  n_bits=24  bin_pt=22  float_type=Single  exp_bits=8  fraction_bits=24  quantization=Truncate  overflow=Flag as error  en=off  latency=0  dbl_ovrd=off  pipeline=off  block_type=convert
  DataReg_En : Subsystem
  Mixer : Subsystem
  Register : xbsIndex_r4/Register  init=0  rst=off  en=off  dbl_ovrd=off  block_type=register
  Terminator : Terminator
  Terminator2 : Terminator
  bpf_out : Outport
  mix_q_out : Outport  Port=2
  mix_i_out : Outport  Port=3
  valid_out : Outport  Port=4
  wires:
  Register/1 -> BPF_FPGA/1
  Constant1/1 -> Mixer/3(en)
  Constant2/1 -> Mixer/1(din_q)
  DDS_valid_in/1 -> Mixer/4(dds_valid)
  DDS_cosine_in/1 -> Mixer/5(dds_cosine)
  DDS_msine_in/1 -> Mixer/6(dds_msine)
  BPF_FPGA/3 -> Convert/1
  Convert/1 -> DataReg_En/1(Din)
  DataReg_En/1(Dout) -> Mixer/2(din_i), bpf_out/1
  BPF_FPGA/2 -> DataReg_En/2(en)
  DataReg_En/2(Valid) -> Terminator2/1
  BPF_FPGA/1 -> Terminator/1
  adc_in/1 -> Register/1
  Mixer/1(Q) -> mix_q_out/1
  Mixer/2(I) -> mix_i_out/1
  Mixer/3(valid_out) -> valid_out/1

== system ddc_bpm_476_066/Channel2_tbt/decim35 ==
  Q_in : Inport
  I_in : Inport  Port=2
  Convert1 : xbsIndex_r4/Convert  gui_display_data_type=Fixed-point  arith_type="Signed  (2's comp)"  n_bits=25  bin_pt=23  float_type=Single  exp_bits=8  fraction_bits=24  quantization="Round  (unbiased: +/- Inf)"  overflow=Flag as error  en=off  latency=0  dbl_ovrd=off  pipeline=off  block_type=convert
  Convert2 : xbsIndex_r4/Convert  gui_display_data_type=Fixed-point  arith_type="Signed  (2's comp)"  n_bits=25  bin_pt=23  float_type=Single  exp_bits=8  fraction_bits=24  quantization="Round  (unbiased: +/- Inf)"  overflow=Flag as error  en=off  latency=0  dbl_ovrd=off  pipeline=off  block_type=convert
  "FIR Compiler 6.2 " : xbsIndex_r4/FIR Compiler 6.2   coefficientvector=Hpoly_35.Numerator  coefficient_sets=1  filter_type=Decimation  rate_change_type=Integer  interpolation_rate=1  decimation_rate=decim_factor_poly_35  number_channels=1  ratespecification=Maximum_Possible  sampleperiod=1  hardwareoversamplingrate=1  filter_architecture=Systolic_Multiply_Accumulate  coefficient_reload=off  coefficient_sign=Signed  quantization=Quantize_Only  coefficient_width=16  bestprecision=on  coefficient_fractional_bits=20  coefficient_structure=Inferred  number_paths=2  output_rounding_mode=Full_Precision  output_width=37  optimization_goal=Area  data_has_tlast=Not_Required  m_data_has_tready=off  s_data_has_fifo=off  s_data_has_tuser=Not_Required  m_data_has_tuser=Not_Required  s_config_sync_mode=On_Vector  s_config_method=Single  num_reload_slots=1  has_aclken=off  has_aresetn=off  multi_column_support=Disabled  columnconfig='14'  inter_column_pipe_length=4  data_buffer_type=Automatic  coefficient_buffer_type=Automatic  input_buffer_type=Automatic  output_buffer_type=Automatic  preference_for_other_storage=Automatic  trim_axipin_name=on  passband_min=0.0  passband_max=0.5  stopband_min=0.5  stopband_max=1.0  filter_selection=1  gui_behaviour=Sysgen_GUI  data_sign=Signed  data_width=16  data_fractional_bits=0  wrapper_available=true  ip_wrap_arbitrary_binary_point=true  ip_name=FIR Compiler  ip_version=6.2  dsptool_ready=true  ipcore_usecache=true  ipcore_useipmodelcache=true  ipcore_xco_need_fpga_part=true  port_translation_map={ 'aclken' => 'en', 'aresetn' => 'rst' }  run_core_at_system_period=true  ipcore_fpga_part=xlipgetpartsetting(gcb, {'virtex6', 'xc6vlx75t', '-3', 'ff784'})  structural_sim=false  block_type=fir_compiler_v6_2
      settings: infoedit=Maximum Possible : Maximizes oversampling rate. Abstracted input handshake (no s_data_tvalid) and automatic rate propagation.<br>Hardware Oversampling Rate : Specifies oversampling rate relative to the input sample period. Abstracted input handshake (no s_data_tvalid) and automatic rate propagation.<br>Sample Period : Specifies absolute oversampling rate. No input handshake abstraction (exposes s_data_tvalid) and no rate propagation.
  Reinterpret : xbsIndex_r4/Reinterpret  force_arith_type=off  arith_type=Unsigned  force_bin_pt=off  bin_pt=43  block_type=reinterpret
  Reinterpret1 : xbsIndex_r4/Reinterpret  force_arith_type=off  arith_type=Unsigned  force_bin_pt=off  bin_pt=43  block_type=reinterpret
  Terminator : Terminator
  Q_out : Outport
  I_out : Outport  Port=2
  valid_out : Outport  Port=3
  wires:
  Q_in/1 -> "FIR Compiler 6.2 "/1
  "FIR Compiler 6.2 "/2 -> valid_out/1
  Reinterpret/1 -> Convert1/1
  "FIR Compiler 6.2 "/3 -> Reinterpret/1
  Convert1/1 -> Q_out/1
  Reinterpret1/1 -> Convert2/1
  "FIR Compiler 6.2 "/4 -> Reinterpret1/1
  Convert2/1 -> I_out/1
  I_in/1 -> "FIR Compiler 6.2 "/2
  "FIR Compiler 6.2 "/1 -> Terminator/1

== system ddc_bpm_476_066/Channel3_fofb/Analysis ==
  CIC_FOFB : Scope  NumInputPorts=2
      settings: TimeRange=0.00011214  YMin=0.440352~-0.0607492  YMax=0.440353~-0.060745  SaveName=ScopeData4  MaxDataPoints=1000000  SampleInput=on
  CORDIC_FOFB : Scope  NumInputPorts=2
      settings: TimeRange=0.00011214  YMin=0.475054~-10  YMax=0.52506~45  SaveName=ScopeData5  MaxDataPoints=1000000  SampleInput=on
  bpf_ch0_o{5..8} (4 alike) : xbsIndex_r4/Gateway Out  inherit_from_input=on  hdl_port=off  timing_constraint=Data Rate  locs_specified=off  LOCs={}  UseAsDAC=off  DACChannel='1'  block_type=gatewayout
      settings: infoedit="Gateway out block.  Converts Xilinx fixed-point or floating-point type inputs into ouputs of type Simulink integer, single, double, or fixed point.<br><br>Hardware notes:  In hardware these blocks become top level output ports or are discarded, depending on how they are configured."
  wires:
  bpf_ch0_o5/1 -> CIC_FOFB/1
  [CIC_FOFB_I_FPGA_OUT] -> bpf_ch0_o5/1
  bpf_ch0_o6/1 -> CIC_FOFB/2
  [CIC_FOFB_Q_FPGA_OUT] -> bpf_ch0_o6/1
  bpf_ch0_o7/1 -> CORDIC_FOFB/1
  [CORDIC_FOFB_R_FPGA_OUT] -> bpf_ch0_o7/1
  bpf_ch0_o8/1 -> CORDIC_FOFB/2
  [CORDIC_FOFB_T_FPGA_OUT] -> bpf_ch0_o8/1

== system ddc_bpm_476_066/Channel3_fofb/cic_fofb ==
  Q_in : Inport
  I_in : Inport  Port=2
  Reinterpret : xbsIndex_r4/Reinterpret  force_arith_type=on  arith_type="Signed  (2's comp)"  force_bin_pt=on  bin_pt=23  block_type=reinterpret
  Reinterpret1 : xbsIndex_r4/Reinterpret  force_arith_type=on  arith_type="Signed  (2's comp)"  force_bin_pt=on  bin_pt=23  block_type=reinterpret
  Terminator : Terminator
  Terminator1 : Terminator
  cic_fofb_i : xbsIndex_r4/CIC Compiler 3.0   filter_type=Decimation  number_of_stages=5  differential_delay=2  number_of_channels=1  sample_rate_changes=Fixed  fixed_or_initial_rate=R_fofb  minimum_rate=1113  maximum_rate=1113  ratespecification=Maximum_Possible  sampleperiod=1  hardwareoversamplingrate=1  quantization=Truncation  output_data_width=25  use_xtreme_dsp_slice=on  use_streaming_interface=on  has_aclken=off  has_aresetn=off  has_dout_tready=off  trim_axipin_name=on  gui_behaviour=Sysgen_GUI  input_data_width=18  ip_name=CIC Compiler  ip_version=3.0  dsptool_ready=true  wrapper_available=true  port_translation_map={ 'aclken' => 'en', 'aresetn' => 'rst' }  ipcore_xco_need_fpga_part=true  ipcore_fpga_part=xlipgetpartsetting(gcb, {'virtex7', 'xc7v1500t', '-2', 'fhg1157'})  ipcore_verbose=false  block_type=cic_compiler_v3_0
  cic_fofb_q : xbsIndex_r4/CIC Compiler 3.0   filter_type=Decimation  number_of_stages=5  differential_delay=2  number_of_channels=1  sample_rate_changes=Fixed  fixed_or_initial_rate=R_fofb  minimum_rate=1113  maximum_rate=1113  ratespecification=Maximum_Possible  sampleperiod=1  hardwareoversamplingrate=1  quantization=Truncation  output_data_width=25  use_xtreme_dsp_slice=on  use_streaming_interface=on  has_aclken=off  has_aresetn=off  has_dout_tready=off  trim_axipin_name=on  gui_behaviour=Sysgen_GUI  input_data_width=18  ip_name=CIC Compiler  ip_version=3.0  dsptool_ready=true  wrapper_available=true  port_translation_map={ 'aclken' => 'en', 'aresetn' => 'rst' }  ipcore_xco_need_fpga_part=true  ipcore_fpga_part=xlipgetpartsetting(gcb, {'virtex7', 'xc7v1500t', '-2', 'fhg1157'})  ipcore_verbose=false  block_type=cic_compiler_v3_0
  Q_out : Outport
  Q_valid : Outport  Port=2
  I_out : Outport  Port=3
  I_valid : Outport  Port=4
  wires:
  I_in/1 -> cic_fofb_i/1
  cic_fofb_i/2 -> I_valid/1
  Q_in/1 -> cic_fofb_q/1
  cic_fofb_q/2 -> Q_valid/1
  cic_fofb_i/1 -> Terminator/1
  cic_fofb_q/1 -> Terminator1/1
  Reinterpret/1 -> Q_out/1
  cic_fofb_q/3 -> Reinterpret/1
  Reinterpret1/1 -> I_out/1
  cic_fofb_i/3 -> Reinterpret1/1
